simulink model "sampleModel1515"  (R2023a)
settings: Solver=VariableStepAuto  StartTime=0.0  StopTime=10.0  RelTol=1e-3
libraries: hdlsllib x7, simulink x3
settings Model: Creator=user1  LastModifiedBy=user1

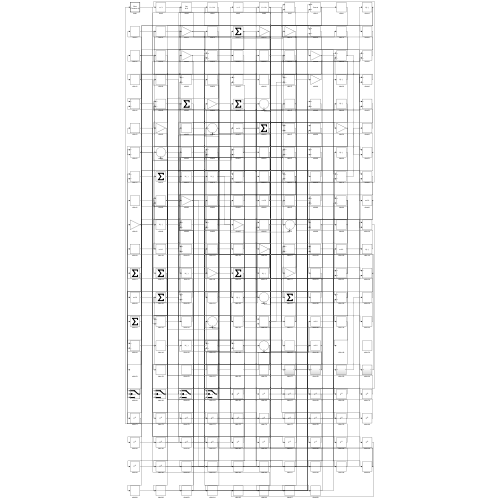
[thumbnail: Simulink's stored preview of the top-level diagram]
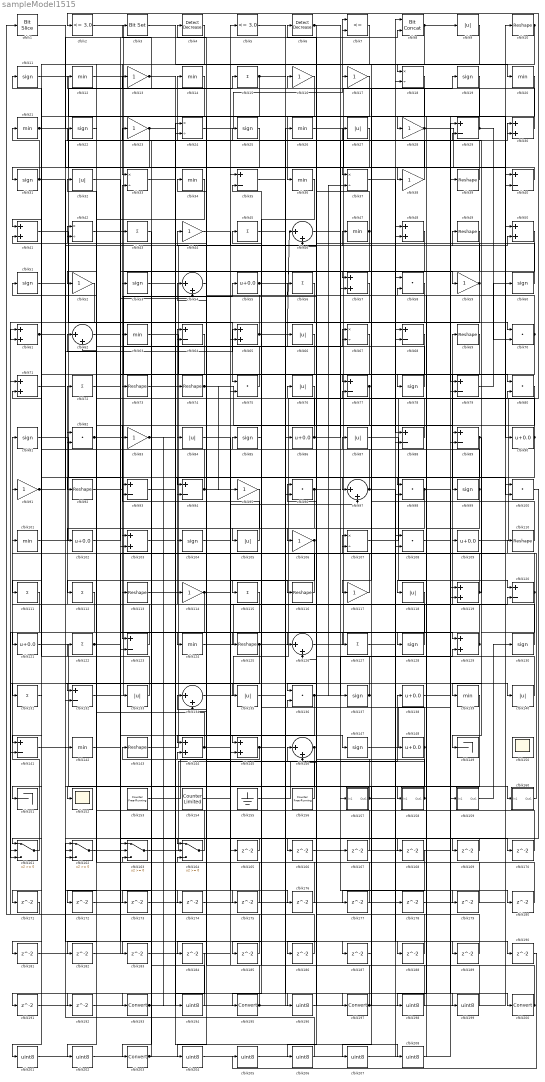
== system sampleModel1515 ==
  cfblk1 : hdlsllib/Logic and Bit Operations/Bit Slice  lidx=7  ridx=0
  cfblk{10,39,49,69,73..74,92,110,113,116,125,143} (12 alike) : Reshape
  cfblk{58,70,75,80,82,96,98,100,108,136} (10 alike) : DotProduct  OutDataTypeStr=Inherit: Inherit via internal rule
  cfblk{12,14,20..21,26,34,36,47,63,101,124,139,142} (13 alike) : MinMax
  cfblk{55,86,90,102,109,121,138,148} (8 alike) : Bias  Bias=0.0  SaturateOnIntegerOverflow=off
  cfblk{30,41,48,50,57,61,65,71,103,119,129,144..145} (13 alike) : Sum
  cfblk{11,19,22,25,31,51,53,60,78,81,85,99,104,128,130,137,147} (17 alike) : Signum
  cfblk{9,27,32,66,76,84,87,105,118,133,135,140} (12 alike) : Abs  SaturateOnIntegerOverflow=off
  cfblk{13,16..17,23,28,38,44,52,59,83,91,95,106,114,117} (15 alike) : Gain
  cfblk{18,24,33,37,42,67,107} (7 alike) : Product  Inputs=*/  RndMeth=Zero  SaturateOnIntegerOverflow=on
  cfblk{15,43,45,56,72,111..112,115,122,127,131} (11 alike) : Sum  Inputs=+
  cfblk{29,35,40,64,68,77,79,88..89,93..94,120,123,132,141} (15 alike) : Sum  Inputs=+-
  cfblk{46,54,62,97,126,134,146} (7 alike) : Sum  Inputs=|++
  cfblk149 : Terminator
  cfblk150 : Scope
      settings: Floating=on
  cfblk151 : Terminator
  cfblk152 : Scope
  cfblk153 : hdlsllib/Sources/Counter Free-Running  NumBits=16  tsamp=-1
  cfblk154 : hdlsllib/Sources/Counter Limited  uplimit=7  tsamp=-1
  cfblk155 : Ground
  cfblk156 : hdlsllib/Sources/Counter Free-Running  NumBits=16  tsamp=-1
  cfblk157 : Subsystem
      settings: LibrarySourceBlock=|
      | hdlsllib/Ports &
      | Subsystems/Subsystem
  cfblk158 : Subsystem
      settings: LibrarySourceBlock=|
      | hdlsllib/Ports &
      | Subsystems/Subsystem
  cfblk159 : Subsystem
      settings: LibrarySourceBlock=|
      | hdlsllib/Ports &
      | Subsystems/Subsystem
  cfblk160 : Subsystem
      settings: LibrarySourceBlock=|
      | hdlsllib/Ports &
      | Subsystems/Subsystem
  cfblk{161..164} (4 alike) : Switch  SaturateOnIntegerOverflow=off  InputSameDT=off
  cfblk{165..192} (28 alike) : Delay  SampleTime=1
  cfblk{193,195,197,200,203} (5 alike) : DataTypeConversion  SaturateOnIntegerOverflow=off  RndMeth=Floor
  cfblk{194,196,198..199,201..202,204..208} (11 alike) : DataTypeConversion  OutDataTypeStr=uint8  SaturateOnIntegerOverflow=off  RndMeth=Floor
  cfblk2 : hdlsllib/Logic and Bit Operations/Compare To Constant  relop=<=  const=3.0  OutDataTypeStr=boolean
  cfblk3 : simulink/Logic and Bit Operations/Bit Set  iBit=0
      settings: LibrarySourceBlock=|
      | hdlsllib/Logic and Bit
      | Operations/Bit Set
  cfblk4 : simulink/Logic and Bit Operations/Detect Decrease  vinit=0.0  OutDataTypeStr=boolean
      settings: LibrarySourceBlock=|
      | hdlsllib/Logic and Bit
      | Operations/Detect
      | Decrease
  cfblk5 : hdlsllib/Logic and Bit Operations/Compare To Constant  relop=<=  const=3.0  OutDataTypeStr=boolean
  cfblk6 : simulink/Logic and Bit Operations/Detect Decrease  vinit=0.0  OutDataTypeStr=boolean
      settings: LibrarySourceBlock=|
      | hdlsllib/Logic and Bit
      | Operations/Detect
      | Decrease
  cfblk7 : RelationalOperator  Operator=<=  OutDataTypeStr=boolean  InputSameDT=off
  cfblk8 : hdlsllib/Logic and Bit Operations/Bit Concat  numInputs=2
  wires:
  cfblk126/1 -> cfblk19/1
  cfblk101/1 -> cfblk15/1
  cfblk24/1 -> cfblk18/1
  cfblk56/1 -> cfblk195/1
  cfblk132/1 -> cfblk67/1
  cfblk22/1 -> cfblk158/1(In1)
  cfblk97/1 -> cfblk71/2, cfblk170/1
  cfblk161/1 -> cfblk81/1
  cfblk108/1 -> cfblk200/1
  cfblk87/1 -> cfblk120/1
  cfblk143/1 -> cfblk49/1
  cfblk145/1 -> cfblk143/1, cfblk107/1
  cfblk77/1 -> cfblk123/1, cfblk94/1
  cfblk119/1 -> cfblk64/1, cfblk29/2
  cfblk117/1 -> cfblk34/1
  cfblk106/1 -> cfblk115/1, cfblk152/1
  cfblk79/1 -> cfblk60/1
  cfblk2/1 -> cfblk78/1
  cfblk136/1 -> cfblk144/1, cfblk37/2, cfblk129/2
  cfblk164/1 -> cfblk62/2
  cfblk82/1 -> cfblk55/1, cfblk54/2, cfblk145/2
  cfblk107/1 -> cfblk39/1
  cfblk155/1 -> cfblk138/1
  cfblk148/1 -> cfblk85/1, cfblk162/3
  cfblk20/1 -> cfblk97/1
  cfblk112/1 -> cfblk121/1
  cfblk123/1 -> cfblk72/1
  cfblk55/1 -> cfblk59/1, cfblk70/1
  cfblk51/1 -> cfblk142/1
  cfblk65/1 -> cfblk46/1, cfblk42/1
  cfblk109/1 -> cfblk2/1
  cfblk35/1 -> cfblk197/1
  cfblk23/1 -> cfblk141/1, cfblk175/1
  cfblk160/1(Out1) -> cfblk110/1
  cfblk124/1 -> cfblk69/1
  cfblk39/1 -> cfblk14/1
  cfblk146/1 -> cfblk182/1, cfblk183/1
  cfblk4/1 -> cfblk33/1
  cfblk34/1 -> cfblk132/1
  cfblk92/1 -> cfblk67/2
  cfblk128/1 -> cfblk104/1
  cfblk3/1 -> cfblk20/1
  cfblk63/1 -> cfblk80/1
  cfblk125/1 -> cfblk68/1, cfblk161/3
  cfblk30/1 -> cfblk7/1
  cfblk40/1 -> cfblk37/1
  cfblk70/1 -> cfblk161/1, cfblk41/2
  cfblk94/1 -> cfblk33/2, cfblk97/2
  cfblk32/1 -> cfblk129/1
  cfblk76/1 -> cfblk103/1
  cfblk159/1(Out1) -> cfblk130/1
  cfblk102/1 -> cfblk7/2
  cfblk88/1 -> cfblk63/1
  cfblk162/1 -> cfblk109/1
  cfblk133/1 -> cfblk11/1
  cfblk121/1 -> cfblk140/1
  cfblk61/1 -> cfblk47/1, cfblk187/1
  cfblk8/1 -> cfblk92/1, cfblk9/1, cfblk46/2
  cfblk69/1 -> cfblk99/1
  cfblk110/1 -> cfblk66/1
  cfblk129/1 -> cfblk91/1, cfblk127/1
  cfblk74/1 -> cfblk137/1, cfblk95/1
  cfblk59/1 -> cfblk102/1, cfblk12/1, cfblk173/1
  cfblk154/1 -> cfblk5/1
  cfblk27/1 -> cfblk31/1
  cfblk98/1 -> cfblk105/1, cfblk180/1
  cfblk68/1 -> cfblk111/1
  cfblk157/1(Out1) -> cfblk44/1, cfblk80/2, cfblk190/1
  cfblk96/1 -> cfblk125/1, cfblk179/1
  cfblk50/1 -> cfblk136/1
  cfblk49/1 -> cfblk103/2
  cfblk10/1 -> cfblk117/1, cfblk131/1
  cfblk48/1 -> cfblk203/1
  cfblk52/1 -> cfblk61/2
  cfblk90/1 -> cfblk164/2, cfblk73/1, cfblk204/1
  cfblk137/1 -> cfblk25/1, cfblk27/1
  cfblk113/1 -> cfblk68/2
  cfblk140/1 -> cfblk84/1
  cfblk118/1 -> cfblk145/1
  cfblk45/1 -> cfblk128/1
  cfblk26/1 -> cfblk50/1
  cfblk9/1 -> cfblk106/1
  cfblk53/1 -> cfblk24/1
  cfblk144/1 -> cfblk120/2, cfblk122/1
  cfblk54/1 -> cfblk124/1
  cfblk105/1 -> cfblk83/1
  cfblk85/1 -> cfblk45/1
  cfblk86/1 -> cfblk32/1, cfblk30/2
  cfblk29/1 -> cfblk16/1, cfblk70/2
  cfblk62/1 -> cfblk77/1
  cfblk1/1 -> cfblk38/1
  cfblk89/1 -> cfblk139/1, cfblk98/1, cfblk181/1
  cfblk28/1 -> cfblk90/1, cfblk126/1, cfblk164/1, cfblk3/1
  cfblk44/1 -> cfblk50/2
  cfblk158/1(Out1) -> cfblk53/1, cfblk146/1
  cfblk91/1 -> cfblk30/1, cfblk189/1
  cfblk57/1 -> cfblk132/2
  cfblk16/1 -> cfblk36/1
  cfblk25/1 -> cfblk41/1
  cfblk41/1 -> cfblk75/1
  cfblk66/1 -> cfblk113/1
  cfblk7/1 -> cfblk151/1
  cfblk122/1 -> cfblk82/1, cfblk188/1
  cfblk75/1 -> cfblk23/1
  cfblk21/1 -> cfblk86/1, cfblk8/2
  cfblk31/1 -> cfblk21/1, cfblk135/1
  cfblk134/1 -> cfblk100/1
  cfblk6/1 -> cfblk89/1, cfblk146/2, cfblk126/2
  cfblk12/1 -> cfblk40/2
  cfblk38/1 -> cfblk22/1
  cfblk13/1 -> cfblk100/2, cfblk57/1
  cfblk15/1 -> cfblk134/2, cfblk57/2, cfblk171/1
  cfblk147/1 -> cfblk119/2
  cfblk60/1 -> cfblk13/1
  cfblk18/1 -> cfblk28/1
  cfblk11/1 -> cfblk79/1
  cfblk99/1 -> cfblk118/1, cfblk87/1
  cfblk83/1 -> cfblk160/1(In1), cfblk194/1
  cfblk14/1 -> cfblk52/1
  cfblk120/1 -> cfblk149/1, cfblk101/1
  cfblk47/1 -> cfblk6/1, cfblk186/1
  cfblk115/1 -> cfblk161/2
  cfblk116/1 -> cfblk93/1
  cfblk81/1 -> cfblk133/1
  cfblk138/1 -> cfblk79/2
  cfblk71/1 -> cfblk65/1
  cfblk130/1 -> cfblk96/1
  cfblk104/1 -> cfblk116/1
  cfblk142/1 -> cfblk147/1
  cfblk43/1 -> cfblk193/1
  cfblk37/1 -> cfblk88/1
  cfblk156/1 -> cfblk134/1
  cfblk153/1 -> cfblk75/2
  cfblk67/1 -> cfblk112/1
  cfblk163/1 -> cfblk148/1
  cfblk103/1 -> cfblk114/1
  cfblk114/1 -> cfblk123/2, cfblk176/1
  cfblk42/1 -> cfblk157/1(In1)
  cfblk135/1 -> cfblk26/1
  cfblk78/1 -> cfblk51/1
  cfblk111/1 -> cfblk141/2
  cfblk127/1 -> cfblk88/2
  cfblk84/1 -> cfblk165/1
  cfblk165/1 -> cfblk163/2
  cfblk100/1 -> cfblk166/1
  cfblk166/1 -> cfblk119/1
  cfblk46/1 -> cfblk167/1
  cfblk167/1 -> cfblk64/2
  cfblk72/1 -> cfblk168/1
  cfblk33/1 -> cfblk169/1
  cfblk169/1 -> cfblk162/2
  cfblk170/1 -> cfblk62/1
  cfblk171/1 -> cfblk1/1
  cfblk80/1 -> cfblk172/1
  cfblk172/1 -> cfblk40/1
  cfblk173/1 -> cfblk93/2
  cfblk141/1 -> cfblk174/1
  cfblk174/1 -> cfblk18/2
  cfblk175/1 -> cfblk94/2
  cfblk176/1 -> cfblk82/2
  cfblk139/1 -> cfblk177/1
  cfblk177/1 -> cfblk54/1
  cfblk178/1 -> cfblk89/2
  cfblk179/1 -> cfblk42/2
  cfblk180/1 -> cfblk144/2
  cfblk181/1 -> cfblk65/2
  cfblk182/1 -> cfblk163/1
  cfblk183/1 -> cfblk24/2
  cfblk17/1 -> cfblk184/1
  cfblk36/1 -> cfblk185/1
  cfblk185/1 -> cfblk61/1
  cfblk186/1 -> cfblk71/1
  cfblk187/1 -> cfblk107/2
  cfblk188/1 -> cfblk136/2
  cfblk189/1 -> cfblk77/2
  cfblk131/1 -> cfblk191/1
  cfblk191/1 -> cfblk10/1
  cfblk95/1 -> cfblk192/1
  cfblk192/1 -> cfblk74/1
  cfblk193/1 -> cfblk178/1, cfblk96/2
  cfblk194/1 -> cfblk43/1
  cfblk195/1 -> cfblk98/2, cfblk4/1
  cfblk73/1 -> cfblk196/1
  cfblk196/1 -> cfblk56/1
  cfblk197/1 -> cfblk29/1, cfblk17/1, cfblk76/1
  cfblk19/1 -> cfblk198/1
  cfblk198/1 -> cfblk35/1
  cfblk5/1 -> cfblk199/1
  cfblk199/1 -> cfblk35/2
  cfblk200/1 -> cfblk164/3, cfblk8/1
  cfblk184/1 -> cfblk201/1
  cfblk201/1 -> cfblk108/1
  cfblk64/1 -> cfblk202/1
  cfblk202/1 -> cfblk108/2
  cfblk203/1 -> cfblk159/1(In1), cfblk163/3
  cfblk204/1 -> cfblk48/1
  cfblk190/1 -> cfblk205/1
  cfblk205/1 -> cfblk48/2
  cfblk58/1 -> cfblk206/1
  cfblk206/1 -> cfblk162/1
  cfblk168/1 -> cfblk207/1
  cfblk207/1 -> cfblk58/1
  cfblk93/1 -> cfblk208/1
  cfblk208/1 -> cfblk58/2

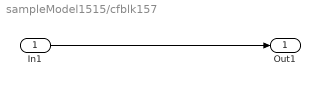
== system sampleModel1515/cfblk157 ==
  In1 : Inport
  Out1 : Outport
  wires:
  In1/1 -> Out1/1

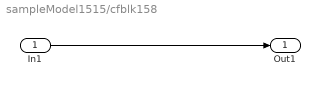
== system sampleModel1515/cfblk158 ==
  In1 : Inport
  Out1 : Outport
  wires:
  In1/1 -> Out1/1

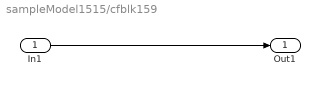
== system sampleModel1515/cfblk159 ==
  In1 : Inport
  Out1 : Outport
  wires:
  In1/1 -> Out1/1

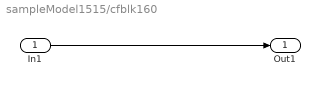
== system sampleModel1515/cfblk160 ==
  In1 : Inport
  Out1 : Outport
  wires:
  In1/1 -> Out1/1
